simulink model "navigation"  (R2021b)
settings: Solver=VariableStepAuto  StartTime=0.0  StopTime=inf  FixedStep=0.001  RelTol=1e-3
model workspace (MAT data in the model file):
  enableTransmit = 1
undefined symbols (not defined in the file or in its folder): sampleTime
libraries: aerolibconvert2 x6, matrix_library x5, sharedutil x4, instrumentlib x1, simulink x1, aerolibutil x1
settings Model: Creator=Vladik  LastModifiedBy=Vladik

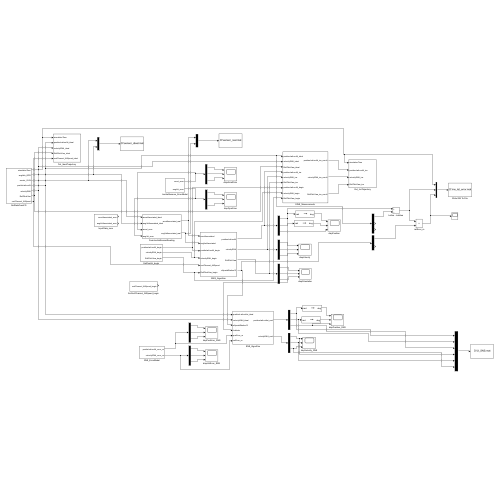
[thumbnail: Simulink's stored preview of the top-level diagram]
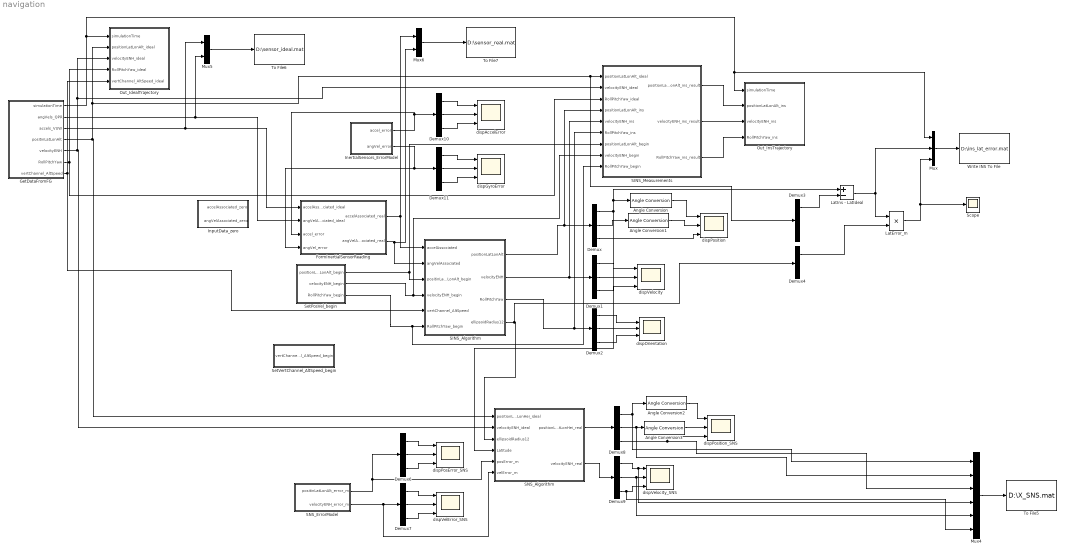
== system navigation ==
  Angle Conversion{,1..3} (4 alike) : aerolibconvert2/Angle Conversion  IU=rad  OU=deg
  Demux{,1..3,6..11} (10 alike) : Demux  Outputs=3
  Demux4 : Demux  Outputs=2
  FormInertialSensorReading : Subsystem
  GetDataFromFG : Subsystem
  InertialSensors_ErrorModel : Subsystem
  InputData_zero : Subsystem
  LatError_m : Product
  LatIns - LatIdeal : Sum  Inputs=+-
  Mux : Mux  Inputs=3
  Mux4 : Mux  Inputs=6
  Mux5 : Mux  Inputs=2
  Mux6 : Mux  Inputs=2
  Out_IdealTrajectory : Subsystem
  Out_InsTrajectory : Subsystem
  SINS_Algorithm : Subsystem
  SINS_Measurements : Subsystem
  SNS_Algorithm : Subsystem
  SNS_ErrorModel : Subsystem
  Scope : Scope
  SetPosVel_begin : Subsystem
  SetVertChannel_AltSpeed_begin : Subsystem
  To File5 : ToFile  Filename=D:\X_SNS.mat  MatrixName=x_sns
  To File6 : ToFile  Filename=D:\sensor_ideal.mat  MatrixName=sensor_ideal
  To File7 : ToFile  Filename=D:\sensor_real.mat  MatrixName=sensor_real
  Write INS To File : ToFile  Filename=D:\ins_lat_error.mat  MatrixName=ins_lat_error
  dispAccelError : Scope  NumInputPorts=3
  dispGyroError : Scope  NumInputPorts=3
  dispOrientation : Scope  NumInputPorts=3
  dispPosError_SNS : Scope  NumInputPorts=3
  dispPosition : Scope  NumInputPorts=3
  dispPosition_SNS : Scope  NumInputPorts=3
  dispVelError_SNS : Scope  NumInputPorts=3
  dispVelocity : Scope  NumInputPorts=3
  dispVelocity_SNS : Scope  NumInputPorts=3
  wires:
  Demux/1 -> LatIns - LatIdeal/1, Angle Conversion/1, SNS_Algorithm/4(Latitude)
  Demux/2 -> Angle Conversion1/1
  Demux1/1 -> dispVelocity/1
  Demux1/2 -> dispVelocity/2
  Demux1/3 -> dispVelocity/3
  Demux2/2 -> dispOrientation/2
  Demux2/1 -> dispOrientation/1
  Demux2/3 -> dispOrientation/3
  GetDataFromFG/4(positinLatLonAlt) -> Out_IdealTrajectory/2(positionLatLonAlt_ideal), Demux3/1, SINS_Measurements/1(positionLatLonAlt_ideal), SNS_Algorithm/1(positionLatLonHei_ideal)
  SINS_Algorithm/1(positionLatLonAlt) -> SINS_Measurements/4(positionLatLonAlt_ins), Demux/1
  SINS_Algorithm/2(velocityENH) -> SINS_Measurements/5(velocityENH_ins), Demux1/1
  SINS_Algorithm/3(RollPitchYaw) -> SINS_Measurements/6(RollPitchYaw_ins), Demux2/1
  SetPosVel_begin/2(velocityENH_begin) -> SINS_Measurements/8(velocityENH_begin), SINS_Algorithm/4(velocityENH_begin)
  Angle Conversion/1 -> dispPosition/1
  Angle Conversion1/1 -> dispPosition/2
  Demux6/1 -> dispPosError_SNS/1
  Demux6/2 -> dispPosError_SNS/2
  Demux6/3 -> dispPosError_SNS/3
  Demux7/1 -> dispVelError_SNS/1
  Demux7/2 -> dispVelError_SNS/2
  Demux7/3 -> dispVelError_SNS/3
  SNS_ErrorModel/2(velocityENH_error_m) -> SNS_Algorithm/6(velError_m), Demux7/1
  SNS_ErrorModel/1(positinLatLonAlt_error_m) -> SNS_Algorithm/5(posError_m), Demux6/1
  SINS_Algorithm/4(ellipsoidRadius12) -> Demux4/1, SNS_Algorithm/3(ellipsoidRadius12)
  SNS_Algorithm/1(positionLatLonHei_real) -> Demux8/1
  Demux8/3 -> Mux4/3, dispPosition_SNS/3
  Demux9/2 -> Mux4/5, dispVelocity_SNS/2
  Demux9/1 -> Mux4/4, dispVelocity_SNS/1
  Demux9/3 -> Mux4/6, dispVelocity_SNS/3
  SNS_Algorithm/2(velocityENH_real) -> Demux9/1
  Demux8/1 -> Angle Conversion2/1, Mux4/1
  Angle Conversion2/1 -> dispPosition_SNS/1
  Demux8/2 -> Mux4/2, Angle Conversion3/1
  Angle Conversion3/1 -> dispPosition_SNS/2
  Demux10/1 -> dispAccelError/1
  Demux10/2 -> dispAccelError/2
  Demux10/3 -> dispAccelError/3
  Demux11/3 -> dispGyroError/3
  Demux11/1 -> dispGyroError/1
  Demux11/2 -> dispGyroError/2
  InertialSensors_ErrorModel/1(accel_error) -> FormInertialSensorReading/3(accel_error), Demux10/1
  InertialSensors_ErrorModel/2(angVel_error) -> FormInertialSensorReading/4(angVel_error), Demux11/1
  FormInertialSensorReading/1(accelAssociated_real) -> SINS_Algorithm/1(accelAssociated), Mux6/1
  FormInertialSensorReading/2(angVelAssociated_real) -> Mux6/2, SINS_Algorithm/2(angVelAssociated)
  SetPosVel_begin/3(RollPitchYaw_begin) -> SINS_Measurements/9(RollPitchYaw_begin), SINS_Algorithm/6(RollPitchYaw_begin)
  SetPosVel_begin/1(positionLatLonAlt_begin) -> SINS_Measurements/7(positionLatLonAlt_begin), SINS_Algorithm/3(positinLatLonAlt_begin)
  GetDataFromFG/3(accels_VUW) -> Mux5/1, FormInertialSensorReading/1(accelAssociated_ideal)
  GetDataFromFG/2(angVels_QPR) -> Mux5/2, FormInertialSensorReading/2(angVelAssociated_ideal)
  GetDataFromFG/7(vertChannel_AltSpeed) -> SINS_Algorithm/5(vertChannel_AltSpeed), Out_IdealTrajectory/5(vertChannel_AltSpeed_ideal)
  GetDataFromFG/5(velocityENH) -> Out_IdealTrajectory/3(velocityENH_ideal), SINS_Measurements/2(velocityENH_ideal), SNS_Algorithm/2(velocityENH_ideal)
  Demux/3 -> dispPosition/3
  Mux4/1 -> To File5/1
  Mux5/1 -> To File6/1
  Mux6/1 -> To File7/1
  GetDataFromFG/6(RollPitchYaw) -> SINS_Measurements/3(RollPitchYaw_ideal), Out_IdealTrajectory/4(RollPitchYaw_ideal)
  SINS_Measurements/2(velocityENH_ins_result) -> Out_InsTrajectory/3(velocityENH_ins)
  SINS_Measurements/3(RollPitchYaw_ins_result) -> Out_InsTrajectory/4(RollPitchYaw_ins)
  SINS_Measurements/1(positionLatLonAlt_ins_result) -> Out_InsTrajectory/2(positionLatLonAlt_ins)
  Demux3/1 -> LatIns - LatIdeal/2
  LatIns - LatIdeal/1 -> Mux/2, LatError_m/1
  Demux4/1 -> LatError_m/2
  GetDataFromFG/1(simulationTime) -> Mux/1, Out_InsTrajectory/1(simulationTime), Out_IdealTrajectory/1(simulationTime)
  Mux/1 -> Write INS To File/1
  LatError_m/1 -> Scope/1, Mux/3

== system navigation/FormInertialSensorReading ==
  accelAssociated_ideal : Inport
  angVelAssociated_ideal : Inport  Port=2
  accel_error : Inport  Port=3
  angVel_error : Inport  Port=4
  Add : Sum
  Add1 : Sum
  accelAssociated_real : Outport
  angVelAssociated_real : Outport  Port=2
  wires:
  accelAssociated_ideal/1 -> Add/1
  accel_error/1 -> Add/2
  Add/1 -> accelAssociated_real/1
  Add1/1 -> angVelAssociated_real/1
  angVelAssociated_ideal/1 -> Add1/1
  angVel_error/1 -> Add1/2

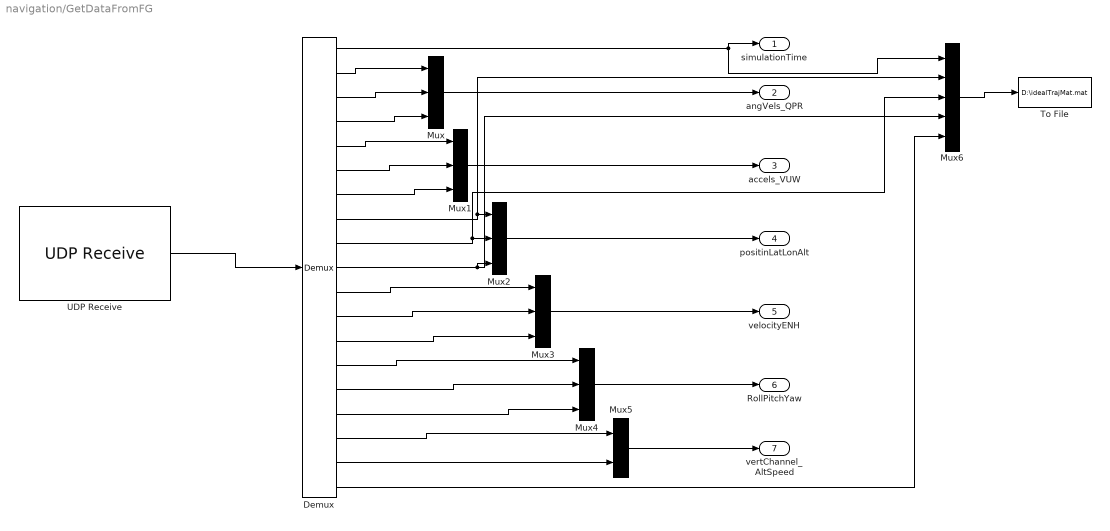
== system navigation/GetDataFromFG ==
  Demux : Demux  Outputs=19
  Mux{,1..4} (5 alike) : Mux  Inputs=3
  Mux5 : Mux  Inputs=2
  Mux6 : Mux  Inputs=5
  To File : ToFile  Filename=D:\idealTrajMat.mat  MatrixName=idealTrajData
  UDP Receive : instrumentlib/UDP Receive  Host=localhost  Port=10000  LocalPort=10000  EnablePortSharing=off  GetLatestData=off  DataSize="[1  19]"  DataType=ASCII  ASCIIFormatting=%f %f %f %f %f %f %f %f %f %f %f %f %f %f %f %f %f %f %f  Terminator=LF  ByteOrder=BigEndian  EnableBlockingMode=on  Timeout=10  SampleTime=0.01  LocalAddress=localhost
  simulationTime : Outport
  angVels_QPR : Outport  Port=2
  accels_VUW : Outport  Port=3
  positinLatLonAlt : Outport  Port=4
  velocityENH : Outport  Port=5
  RollPitchYaw : Outport  Port=6
  vertChannel_AltSpeed : Outport  Port=7
  wires:
  UDP Receive/1 -> Demux/1
  Demux/2 -> Mux/1
  Demux/3 -> Mux/2
  Demux/4 -> Mux/3
  Demux/5 -> Mux1/1
  Demux/6 -> Mux1/2
  Demux/7 -> Mux1/3
  Demux/8 -> Mux6/2, Mux2/1
  Demux/9 -> Mux6/3, Mux2/2
  Demux/10 -> Mux2/3, Mux6/4
  Mux/1 -> angVels_QPR/1
  Mux1/1 -> accels_VUW/1
  Mux2/1 -> positinLatLonAlt/1
  Demux/11 -> Mux3/1
  Demux/12 -> Mux3/2
  Demux/13 -> Mux3/3
  Mux3/1 -> velocityENH/1
  Demux/14 -> Mux4/1
  Demux/15 -> Mux4/2
  Demux/16 -> Mux4/3
  Mux4/1 -> RollPitchYaw/1
  Demux/17 -> Mux5/1
  Demux/18 -> Mux5/2
  Mux5/1 -> vertChannel_AltSpeed/1
  Demux/1 -> simulationTime/1, Mux6/1
  Mux6/1 -> To File/1
  Demux/19 -> Mux6/5

== system navigation/InertialSensors_ErrorModel ==
  Add{,1..5} (6 alike) : Sum
  Mux : Mux  Inputs=3
  Mux1 : Mux  Inputs=3
  Ramp : simulink/Sources/Ramp  slope=0.15*pi/180/3600  start=0  InitialOutput=0
  accelNoise : RandomNumber  Mean=1e-6  Variance=0  SampleTime=1
  accelZeroOffset : Constant  Value=0.005
  gyroNoise : RandomNumber  Mean=(0.1*pi/180/3600)^2  Variance=0  SampleTime=1
  accel_error : Outport
  angVel_error : Outport  Port=2
  wires:
  gyroNoise/1 -> Add/2, Add5/2, Add4/2
  accelZeroOffset/1 -> Add2/1, Add3/1, Add1/1
  accelNoise/1 -> Add3/2, Add2/2, Add1/2
  Add1/1 -> Mux/2
  Mux/1 -> accel_error/1
  Mux1/1 -> angVel_error/1
  Add2/1 -> Mux/1
  Add3/1 -> Mux/3
  Ramp/1 -> Add5/1, Add4/1, Add/1
  Add4/1 -> Mux1/2
  Add/1 -> Mux1/1
  Add5/1 -> Mux1/3

== system navigation/InputData_zero ==
  Constant : Constant  Value=1e-5
  Constant1 : Constant  Value=1e-5
  Constant2 : Constant  Value=0.1
  Mux : Mux  Inputs=3
  Mux1 : Mux  Inputs=3
  accelAssociated_zero : Outport
  angVelAssociated_zero : Outport  Port=2
  wires:
  Constant/1 -> Mux1/2, Mux1/3, Mux1/1, Mux/2
  Mux/1 -> accelAssociated_zero/1
  Mux1/1 -> angVelAssociated_zero/1
  Constant1/1 -> Mux/3
  Constant2/1 -> Mux/1

== system navigation/Out_IdealTrajectory ==
  simulationTime : Inport
  positionLatLonAlt_ideal : Inport  Port=2
  velocityENH_ideal : Inport  Port=3
  RollPitchYaw_ideal : Inport  Port=4
  vertChannel_AltSpeed_ideal : Inport  Port=5
  Demux3 : Demux  Outputs=3
  Demux4 : Demux  Outputs=3
  Demux5 : Demux  Outputs=3
  Vector Concatenate2 : Concatenate  NumInputs=5  Mode=Multidimensional array
  Write Ideal To File : ToFile  Filename=D:\x_ideal.mat  MatrixName=x_ideal
  dispOrientationIdeal : Scope  NumInputPorts=3
  dispPositionIdeal : Scope  NumInputPorts=3
  dispVelocityIdeal : Scope  NumInputPorts=3
  wires:
  simulationTime/1 -> Vector Concatenate2/1
  positionLatLonAlt_ideal/1 -> Demux3/1, Vector Concatenate2/2
  RollPitchYaw_ideal/1 -> Demux5/1, Vector Concatenate2/4
  vertChannel_AltSpeed_ideal/1 -> Vector Concatenate2/5
  Vector Concatenate2/1 -> Write Ideal To File/1
  Demux3/2 -> dispPositionIdeal/2
  Demux3/3 -> dispPositionIdeal/3
  Demux3/1 -> dispPositionIdeal/1
  velocityENH_ideal/1 -> Demux4/1, Vector Concatenate2/3
  Demux4/1 -> dispVelocityIdeal/1
  Demux4/2 -> dispVelocityIdeal/2
  Demux4/3 -> dispVelocityIdeal/3
  Demux5/3 -> dispOrientationIdeal/3
  Demux5/2 -> dispOrientationIdeal/2
  Demux5/1 -> dispOrientationIdeal/1

== system navigation/Out_InsTrajectory ==
  simulationTime : Inport
  positionLatLonAlt_ins : Inport  Port=2
  velocityENH_ins : Inport  Port=3
  RollPitchYaw_ins : Inport  Port=4
  Demux3 : Demux  Outputs=3
  Demux4 : Demux  Outputs=3
  Demux5 : Demux  Outputs=3
  Vector Concatenate2 : Concatenate  NumInputs=4  Mode=Multidimensional array
  Write INS To File : ToFile  Filename=D:\x_ins.mat  MatrixName=x_ins
  dispOrientationINS : Scope  NumInputPorts=3
  dispPositionINS : Scope  NumInputPorts=3
  dispVelocityINS : Scope  NumInputPorts=3
  wires:
  simulationTime/1 -> Vector Concatenate2/1
  positionLatLonAlt_ins/1 -> Demux3/1, Vector Concatenate2/2
  RollPitchYaw_ins/1 -> Demux5/1, Vector Concatenate2/4
  Vector Concatenate2/1 -> Write INS To File/1
  Demux3/2 -> dispPositionINS/2
  Demux3/3 -> dispPositionINS/3
  Demux3/1 -> dispPositionINS/1
  velocityENH_ins/1 -> Demux4/1, Vector Concatenate2/3
  Demux4/1 -> dispVelocityINS/1
  Demux4/2 -> dispVelocityINS/2
  Demux4/3 -> dispVelocityINS/3
  Demux5/3 -> dispOrientationINS/3
  Demux5/2 -> dispOrientationINS/2
  Demux5/1 -> dispOrientationINS/1

== system navigation/SINS_Algorithm ==
  accelAssociated : Inport
  angVelAssociated : Inport  Port=2
  positinLatLonAlt_begin : Inport  Port=3
  velocityENH_begin : Inport  Port=4
  vertChannel_AltSpeed : Inport  Port=5
  RollPitchYaw_begin : Inport  Port=6
  CalculateAccelerationsXYZ : Subsystem
  GetC_begin : Subsystem  Commented=on
  GetC_begin_easy : Subsystem
  NavigationAlgorithm : Subsystem
  OrientationAlgorithm : Subsystem
  U_earth : Constant  Value=7.29212e-5
  removeVelocityH : Subsystem
  positionLatLonAlt : Outport
  velocityENH : Outport  Port=2
  RollPitchYaw : Outport  Port=3
  ellipsoidRadius12 : Outport  Port=4
  wires:
  accelAssociated/1 -> CalculateAccelerationsXYZ/1(accelerationAssociated)
  OrientationAlgorithm/1(C_assoc_norm) -> CalculateAccelerationsXYZ/2(C_accoc_norm)
  angVelAssociated/1 -> OrientationAlgorithm/1(angVel_inertial_assoc)
  NavigationAlgorithm/3(angVelNorm_matrix_3x3) -> OrientationAlgorithm/2(angVelNorm_matrix)
  NavigationAlgorithm/1(positionLatLonAlt) -> positionLatLonAlt/1
  NavigationAlgorithm/2(velocityENH) -> velocityENH/1
  OrientationAlgorithm/2(RollPitchYaw) -> RollPitchYaw/1
  positinLatLonAlt_begin/1 -> NavigationAlgorithm/2(positionLatLonAlt_begin)
  U_earth/1 -> NavigationAlgorithm/4(U_earth)
  vertChannel_AltSpeed/1 -> NavigationAlgorithm/5(vertChannel_AltSpeed)
  NavigationAlgorithm/4(ellipsoidRadius12) -> ellipsoidRadius12/1
  velocityENH_begin/1 -> removeVelocityH/1(velocityENH_begin)
  removeVelocityH/1(velocityEN_begin) -> NavigationAlgorithm/3(velocityEN_begin)
  RollPitchYaw_begin/1 -> GetC_begin_easy/1(RollPitchYaw_begin)
  GetC_begin_easy/1(C_assoc_norm_begin) -> OrientationAlgorithm/3(C_assoc_norm_begin)
  CalculateAccelerationsXYZ/1(accelerationXYZ) -> NavigationAlgorithm/1(accelerationXYZ)

== system navigation/SINS_Measurements ==
  positionLatLonAlt_ideal : Inport
  velocityENH_ideal : Inport  Port=2
  RollPitchYaw_ideal : Inport  Port=3
  positionLatLonAlt_ins : Inport  Port=4
  velocityENH_ins : Inport  Port=5
  RollPitchYaw_ins : Inport  Port=6
  positionLatLonAlt_begin : Inport  Port=7
  velocityENH_begin : Inport  Port=8
  RollPitchYaw_begin : Inport  Port=9
  Subtract1 : Sum  Inputs=++-
  Subtract2 : Sum  Inputs=++-
  Subtract3 : Sum  Inputs=++-
  positionLatLonAlt_ins_result : Outport
  velocityENH_ins_result : Outport  Port=2
  RollPitchYaw_ins_result : Outport  Port=3
  wires:
  positionLatLonAlt_ideal/1 -> Subtract3/1
  positionLatLonAlt_ins/1 -> Subtract3/2
  positionLatLonAlt_begin/1 -> Subtract3/3
  velocityENH_ideal/1 -> Subtract1/1
  velocityENH_ins/1 -> Subtract1/2
  velocityENH_begin/1 -> Subtract1/3
  RollPitchYaw_ideal/1 -> Subtract2/1
  RollPitchYaw_ins/1 -> Subtract2/2
  RollPitchYaw_begin/1 -> Subtract2/3
  Subtract3/1 -> positionLatLonAlt_ins_result/1
  Subtract1/1 -> velocityENH_ins_result/1
  Subtract2/1 -> RollPitchYaw_ins_result/1

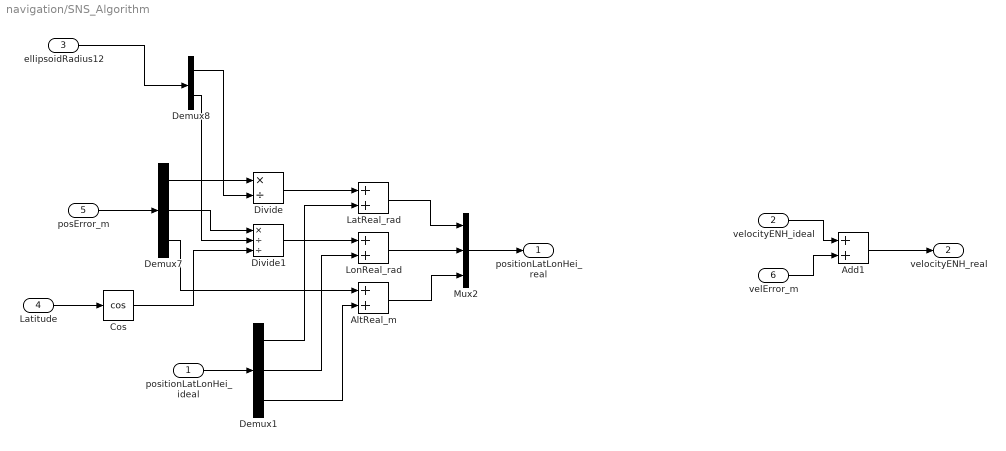
== system navigation/SNS_Algorithm ==
  positionLatLonHei_ideal : Inport
  velocityENH_ideal : Inport  Port=2
  ellipsoidRadius12 : Inport  Port=3
  Latitude : Inport  Port=4
  posError_m : Inport  Port=5
  velError_m : Inport  Port=6
  Add1 : Sum
  AltReal_m : Sum
  Cos : Trigonometry  Operator=cos
  Demux1 : Demux  Outputs=3
  Demux7 : Demux  Outputs=3
  Demux8 : Demux  Outputs=2
  Divide : Product  Inputs=*/
  Divide1 : Product  Inputs=*//
  LatReal_rad : Sum
  LonReal_rad : Sum
  Mux2 : Mux  Inputs=3
  positionLatLonHei_real : Outport
  velocityENH_real : Outport  Port=2
  wires:
  Divide1/1 -> LonReal_rad/1
  Divide/1 -> LatReal_rad/1
  ellipsoidRadius12/1 -> Demux8/1
  posError_m/1 -> Demux7/1
  Demux7/1 -> Divide/1
  Demux8/1 -> Divide/2
  Demux7/2 -> Divide1/1
  Demux8/2 -> Divide1/2
  Latitude/1 -> Cos/1
  Cos/1 -> Divide1/3
  positionLatLonHei_ideal/1 -> Demux1/1
  Demux1/1 -> LatReal_rad/2
  Demux1/2 -> LonReal_rad/2
  Demux7/3 -> AltReal_m/1
  Demux1/3 -> AltReal_m/2
  LonReal_rad/1 -> Mux2/2
  LatReal_rad/1 -> Mux2/1
  AltReal_m/1 -> Mux2/3
  Mux2/1 -> positionLatLonHei_real/1
  velocityENH_ideal/1 -> Add1/1
  velError_m/1 -> Add1/2
  Add1/1 -> velocityENH_real/1

== system navigation/SNS_ErrorModel ==
  AltError_m : RandomNumber  Variance=225  SampleTime=sampleTime
  LatError_m : RandomNumber  Variance=225  SampleTime=sampleTime
  LonError_m : RandomNumber  Variance=225  SampleTime=sampleTime
  Mux : Mux  Inputs=3
  Mux1 : Mux  Inputs=3
  VelE_error_m : RandomNumber  Variance=0.01  SampleTime=sampleTime
  VelH_error_m : RandomNumber  Variance=0.01  SampleTime=sampleTime
  VelN_error_m : RandomNumber  Variance=0.01  SampleTime=sampleTime
  positinLatLonAlt_error_m : Outport
  velocityENH_error_m : Outport  Port=2
  wires:
  LonError_m/1 -> Mux/2
  LatError_m/1 -> Mux/1
  AltError_m/1 -> Mux/3
  Mux/1 -> positinLatLonAlt_error_m/1
  VelN_error_m/1 -> Mux1/2
  VelE_error_m/1 -> Mux1/1
  VelH_error_m/1 -> Mux1/3
  Mux1/1 -> velocityENH_error_m/1

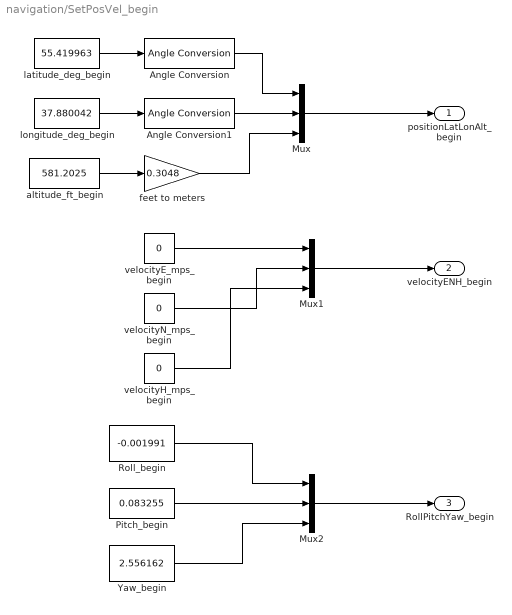
== system navigation/SetPosVel_begin ==
  Angle Conversion : aerolibconvert2/Angle Conversion  IU=deg  OU=rad
  Angle Conversion1 : aerolibconvert2/Angle Conversion  IU=deg  OU=rad
  Mux : Mux  Inputs=3
  Mux1 : Mux  Inputs=3
  Mux2 : Mux  Inputs=3
  Pitch_begin : Constant  Value=0.083255
  Roll_begin : Constant  Value=-0.001991
  Yaw_begin : Constant  Value=2.556162
  altitude_ft_begin : Constant  Value=581.2025
  feet to meters : Gain  Gain=0.3048
  latitude_deg_begin : Constant  Value=55.419963
  longitude_deg_begin : Constant  Value=37.880042
  velocityE_mps_begin : Constant  Value=0
  velocityH_mps_begin : Constant  Value=0
  velocityN_mps_begin : Constant  Value=0
  positionLatLonAlt_begin : Outport
  velocityENH_begin : Outport  Port=2
  RollPitchYaw_begin : Outport  Port=3
  wires:
  altitude_ft_begin/1 -> feet to meters/1
  latitude_deg_begin/1 -> Angle Conversion/1
  Mux1/1 -> velocityENH_begin/1
  velocityE_mps_begin/1 -> Mux1/1
  Angle Conversion1/1 -> Mux/2
  feet to meters/1 -> Mux/3
  velocityN_mps_begin/1 -> Mux1/2
  longitude_deg_begin/1 -> Angle Conversion1/1
  Angle Conversion/1 -> Mux/1
  Mux/1 -> positionLatLonAlt_begin/1
  velocityH_mps_begin/1 -> Mux1/3
  Yaw_begin/1 -> Mux2/3
  Pitch_begin/1 -> Mux2/2
  Roll_begin/1 -> Mux2/1
  Mux2/1 -> RollPitchYaw_begin/1

== system navigation/SetVertChannel_AltSpeed_begin ==
  Mux : Mux  Inputs=2
  altitude_ft_begin : Constant  Value=497.4182917
  feet to meters : Gain  Gain=0.3048
  velocityH_mps_begin : Constant  Value=0
  vertChannel_AltSpeed_begin : Outport
  wires:
  velocityH_mps_begin/1 -> Mux/2
  feet to meters/1 -> Mux/1
  altitude_ft_begin/1 -> feet to meters/1
  Mux/1 -> vertChannel_AltSpeed_begin/1

== system navigation/SINS_Algorithm/CalculateAccelerationsXYZ ==
  accelerationAssociated : Inport
  C_accoc_norm : Inport  Port=2
  Product : Product  Multiplication=Matrix(*)
  accelerationXYZ : Outport
  wires:
  accelerationAssociated/1 -> Product/2
  Product/1 -> accelerationXYZ/1
  C_accoc_norm/1 -> Product/1

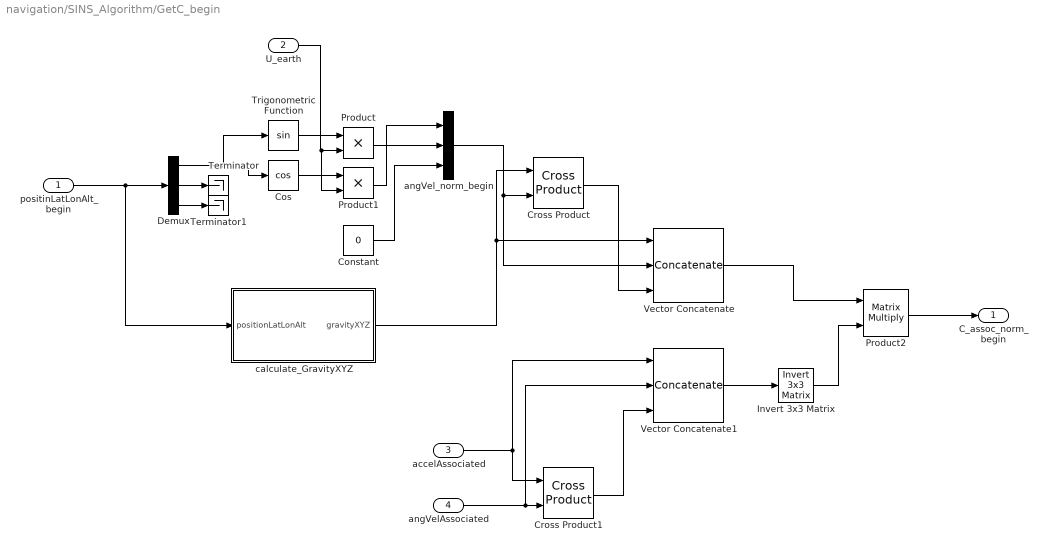
== system navigation/SINS_Algorithm/GetC_begin ==
  positinLatLonAlt_begin : Inport
  U_earth : Inport  Port=2
  accelAssociated : Inport  Port=3
  angVelAssociated : Inport  Port=4
  Constant : Constant  Value=0
  Cos : Trigonometry  Operator=cos
  Cross Product : matrix_library/Cross Product
      settings: SourceProductBaseCode=SL
  Cross Product1 : matrix_library/Cross Product
      settings: SourceProductBaseCode=SL
  Demux : Demux  Outputs=3
  Invert 3x3 Matrix : aerolibutil/Invert  3x3 Matrix
  Product : Product
  Product1 : Product
  Product2 : Product  Multiplication=Matrix(*)
  Terminator : Terminator
  Terminator1 : Terminator
  Trigonometric Function : Trigonometry
  Vector Concatenate : Concatenate  NumInputs=3  Mode=Multidimensional array  ConcatenateDimension=2
  Vector Concatenate1 : Concatenate  NumInputs=3  Mode=Multidimensional array  ConcatenateDimension=2
  angVel_norm_begin : Mux  Inputs=3
  calculate_GravityXYZ : Subsystem
  C_assoc_norm_begin : Outport
  wires:
  Trigonometric Function/1 -> Product/1
  Demux/1 -> Cos/1, Trigonometric Function/1
  Cos/1 -> Product1/1
  Constant/1 -> angVel_norm_begin/3
  Product/1 -> angVel_norm_begin/2
  Product1/1 -> angVel_norm_begin/1
  Demux/3 -> Terminator1/1
  Demux/2 -> Terminator/1
  calculate_GravityXYZ/1(gravityXYZ) -> Vector Concatenate/1, Cross Product/1
  angVel_norm_begin/1 -> Vector Concatenate/2, Cross Product/2
  positinLatLonAlt_begin/1 -> calculate_GravityXYZ/1(positionLatLonAlt), Demux/1
  U_earth/1 -> Product1/2, Product/2
  Cross Product/1 -> Vector Concatenate/3
  accelAssociated/1 -> Vector Concatenate1/1, Cross Product1/1
  angVelAssociated/1 -> Vector Concatenate1/2, Cross Product1/2
  Cross Product1/1 -> Vector Concatenate1/3
  Vector Concatenate1/1 -> Invert 3x3 Matrix/1
  Vector Concatenate/1 -> Product2/1
  Invert 3x3 Matrix/1 -> Product2/2
  Product2/1 -> C_assoc_norm_begin/1

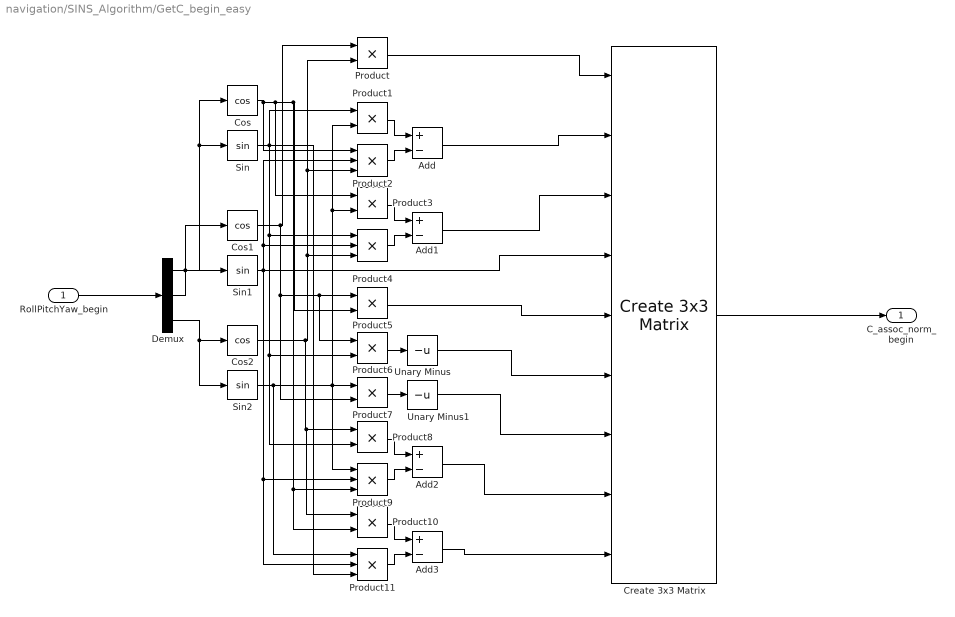
== system navigation/SINS_Algorithm/GetC_begin_easy ==
  RollPitchYaw_begin : Inport
  Add{,1..3} (4 alike) : Sum  Inputs=+-
  Cos : Trigonometry  Operator=cos
  Cos1 : Trigonometry  Operator=cos
  Cos2 : Trigonometry  Operator=cos
  Create 3x3 Matrix : sharedutil/Create 3x3 Matrix  aMode=aMode
      settings: SourceProductBaseCode=AE,PW,DR,MT,UV,VE
  Demux : Demux  Outputs=3
  Product{,1,3,5..8,10} (8 alike) : Product
  Product{2,4,9,11} (4 alike) : Product  Inputs=3
  Sin : Trigonometry
  Sin1 : Trigonometry
  Sin2 : Trigonometry
  Unary Minus : UnaryMinus
  Unary Minus1 : UnaryMinus
  C_assoc_norm_begin : Outport
  wires:
  RollPitchYaw_begin/1 -> Demux/1
  Demux/1 -> Sin/1, Cos/1
  Demux/2 -> Sin1/1, Cos1/1
  Demux/3 -> Sin2/1, Cos2/1
  Cos1/1 -> Product7/2, Product6/1, Product5/1, Product/1
  Sin2/1 -> Product11/1, Product9/1, Product7/1, Product3/2, Product1/2
  Sin/1 -> Product11/3, Product8/2, Product6/2, Product4/1, Product1/1
  Sin1/1 -> Product11/2, Product9/2, Create 3x3 Matrix/4, Product4/2, Product2/2
  Cos/1 -> Product10/2, Product9/3, Product5/2, Product3/1, Product2/1
  Product1/1 -> Add/1
  Product2/1 -> Add/2
  Product/1 -> Create 3x3 Matrix/1
  Add/1 -> Create 3x3 Matrix/2
  Product4/1 -> Add1/2
  Product3/1 -> Add1/1
  Add1/1 -> Create 3x3 Matrix/3
  Product5/1 -> Create 3x3 Matrix/5
  Product6/1 -> Unary Minus/1
  Unary Minus/1 -> Create 3x3 Matrix/6
  Product7/1 -> Unary Minus1/1
  Cos2/1 -> Product10/1, Product8/1, Product4/3, Product2/3, Product/2
  Unary Minus1/1 -> Create 3x3 Matrix/7
  Product8/1 -> Add2/1
  Product9/1 -> Add2/2
  Add2/1 -> Create 3x3 Matrix/8
  Product11/1 -> Add3/2
  Product10/1 -> Add3/1
  Add3/1 -> Create 3x3 Matrix/9
  Create 3x3 Matrix/1 -> C_assoc_norm_begin/1

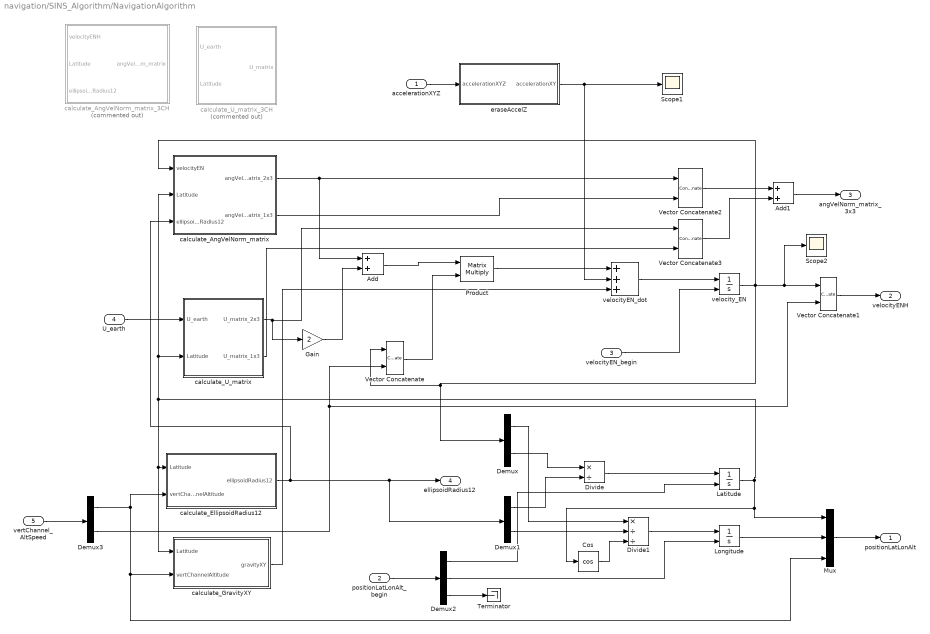
== system navigation/SINS_Algorithm/NavigationAlgorithm ==
  accelerationXYZ : Inport
  positionLatLonAlt_begin : Inport  Port=2
  velocityEN_begin : Inport  Port=3
  U_earth : Inport  Port=4
  vertChannel_AltSpeed : Inport  Port=5
  Add : Sum
  Add1 : Sum
  Cos : Trigonometry  Operator=cos
  Demux : Demux  Outputs=2
  Demux1 : Demux  Outputs=2
  Demux2 : Demux  Outputs=3
  Demux3 : Demux  Outputs=2
  Divide : Product  Inputs=*/
  Divide1 : Product  Inputs=*//
  Gain : Gain  Gain=2
  Latitude : Integrator  InitialConditionSource=external
  Longitude : Integrator  InitialConditionSource=external
  Mux : Mux  Inputs=3
  Product : Product  Multiplication=Matrix(*)
  Scope1 : Scope
  Scope2 : Scope
  Terminator : Terminator
  Vector Concatenate{,1..3} (4 alike) : Concatenate  Mode=Multidimensional array
  calculate_AngVelNorm_matrix : Subsystem
  calculate_AngVelNorm_matrix_3CH : Subsystem  Commented=on
  calculate_EllipsoidRadius12 : Subsystem
  calculate_GravityXY : Subsystem
  calculate_U_matrix : Subsystem
  calculate_U_matrix_3CH : Subsystem  Commented=on
  eraseAccelZ : Subsystem
  velocityEN_dot : Sum  Inputs=+++
  velocity_EN : Integrator  InitialConditionSource=external  InitialCondition=[0; 0; 0]
  positionLatLonAlt : Outport
  velocityENH : Outport  Port=2
  angVelNorm_matrix_3x3 : Outport  Port=3
  ellipsoidRadius12 : Outport  Port=4
  wires:
  calculate_U_matrix/1(U_matrix_2x3) -> Vector Concatenate3/1, Gain/1
  calculate_AngVelNorm_matrix/1(angVelNorm_matrix_2x3) -> Vector Concatenate2/1, Add/1
  Gain/1 -> Add/2
  Add/1 -> Product/1
  Product/1 -> velocityEN_dot/1
  velocityEN_dot/1 -> velocity_EN/1
  Divide/1 -> Latitude/1
  Demux/2 -> Divide/1
  Demux1/1 -> Divide/2
  Latitude/1 -> calculate_GravityXY/1(Latitude), calculate_EllipsoidRadius12/1(Latitude), calculate_U_matrix/2(Latitude), calculate_AngVelNorm_matrix/2(Latitude), Mux/1, Cos/1
  Divide1/1 -> Longitude/1
  Demux/1 -> Divide1/1
  Demux1/2 -> Divide1/2
  Cos/1 -> Divide1/3
  Longitude/1 -> Mux/2
  Demux3/1 -> Mux/3, calculate_GravityXY/2(vertChannelAltitude), calculate_EllipsoidRadius12/2(vertChannelAltitude)
  calculate_EllipsoidRadius12/1(ellipsoidRadius12) -> calculate_AngVelNorm_matrix/3(ellipsoidRadius12), ellipsoidRadius12/1, Demux1/1
  U_earth/1 -> calculate_U_matrix/1(U_earth)
  Mux/1 -> positionLatLonAlt/1
  velocity_EN/1 -> Scope2/1, Vector Concatenate1/1, calculate_AngVelNorm_matrix/1(velocityEN), Vector Concatenate/1, Demux/1
  calculate_GravityXY/1(gravityXY) -> velocityEN_dot/3
  positionLatLonAlt_begin/1 -> Demux2/1
  Demux2/1 -> Latitude/2
  Demux2/2 -> Longitude/2
  velocityEN_begin/1 -> velocity_EN/2
  vertChannel_AltSpeed/1 -> Demux3/1
  Demux3/2 -> Vector Concatenate1/2, Vector Concatenate/2
  Vector Concatenate/1 -> Product/2
  Vector Concatenate1/1 -> velocityENH/1
  calculate_AngVelNorm_matrix/2(angVelNorm_matrix_1x3) -> Vector Concatenate2/2
  accelerationXYZ/1 -> eraseAccelZ/1(accelerationXYZ)
  eraseAccelZ/1(accelerationXY) -> Scope1/1, velocityEN_dot/2
  Demux2/3 -> Terminator/1
  calculate_U_matrix/2(U_matrix_1x3) -> Vector Concatenate3/2
  Vector Concatenate2/1 -> Add1/1
  Vector Concatenate3/1 -> Add1/2
  Add1/1 -> angVelNorm_matrix_3x3/1

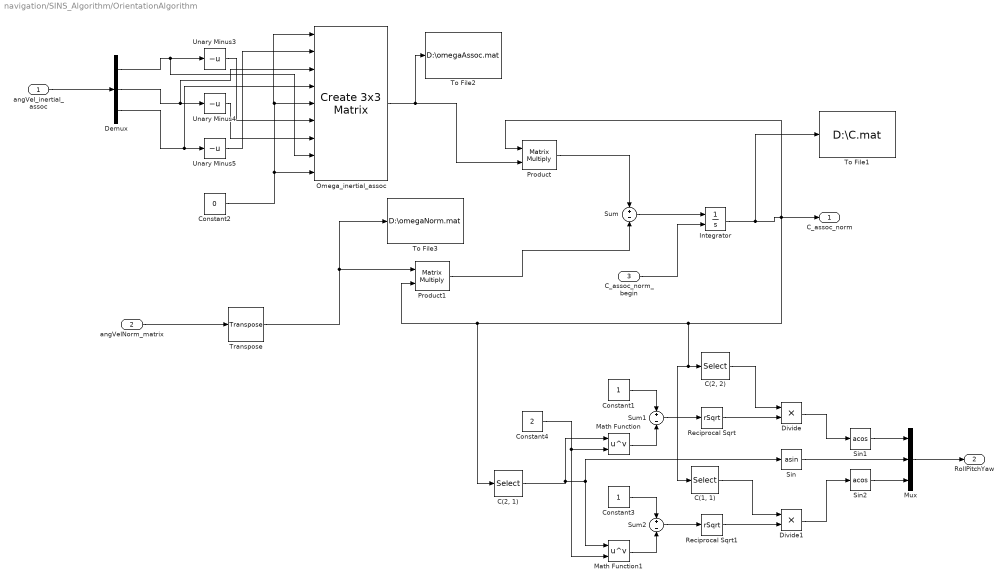
== system navigation/SINS_Algorithm/OrientationAlgorithm ==
  angVel_inertial_assoc : Inport
  angVelNorm_matrix : Inport  Port=2
  C_assoc_norm_begin : Inport  Port=3
  "C(1, 1)" : Selector  NumberOfDimensions=2  InputPortWidth=3  IndexOptions=Index vector (dialog),Index vector (dialog)  Indices=1,1  OutputSizes=1,1
  "C(2, 1)" : Selector  NumberOfDimensions=2  InputPortWidth=3  IndexOptions=Index vector (dialog),Index vector (dialog)  Indices=2,1  OutputSizes=1,1
  "C(2, 2)" : Selector  NumberOfDimensions=2  InputPortWidth=3  IndexOptions=Index vector (dialog),Index vector (dialog)  Indices=2,2  OutputSizes=1,1
  Constant1 : Constant
  Constant2 : Constant  Value=0
  Constant3 : Constant
  Constant4 : Constant  Value=2
  Demux : Demux  Outputs=3
  Divide : Product  Inputs=**
  Divide1 : Product  Inputs=**
  Integrator : Integrator  InitialConditionSource=external  InitialCondition=[0, 0, 0; 0, 0, 0; 0, 0, 0]
  Math Function : Math  Operator=pow  SaturateOnIntegerOverflow=on
  Math Function1 : Math  Operator=pow  SaturateOnIntegerOverflow=on
  Mux : Mux  Inputs=3
  Omega_inertial_assoc : sharedutil/Create 3x3 Matrix  aMode=aMode
      settings: SourceProductBaseCode=AE,PW,DR,MT,UV,VE
  Product : Product  Multiplication=Matrix(*)
  Product1 : Product  Multiplication=Matrix(*)
  Reciprocal Sqrt : Sqrt  Operator=rSqrt  SaturateOnIntegerOverflow=on
  Reciprocal Sqrt1 : Sqrt  Operator=rSqrt  SaturateOnIntegerOverflow=on
  Sin : Trigonometry  Operator=asin
  Sin1 : Trigonometry  Operator=acos
  Sin2 : Trigonometry  Operator=acos
  Sum : Sum  Inputs=+-
  Sum1 : Sum  Inputs=+-
  Sum2 : Sum  Inputs=+-
  To File1 : ToFile  Filename=D:\C.mat  MatrixName=C  SaveFormat=Timeseries
  To File2 : ToFile  Filename=D:\omegaAssoc.mat  MatrixName=omegaAssoc  SaveFormat=Timeseries
  To File3 : ToFile  Filename=D:\omegaNorm.mat  MatrixName=omegaNorm  SaveFormat=Timeseries
  Transpose : matrix_library/Transpose
      settings: SourceProductBaseCode=SL
  Unary Minus3 : UnaryMinus
  Unary Minus4 : UnaryMinus
  Unary Minus5 : UnaryMinus
  C_assoc_norm : Outport
  RollPitchYaw : Outport  Port=2
  wires:
  angVel_inertial_assoc/1 -> Demux/1
  angVelNorm_matrix/1 -> Transpose/1
  Sum/1 -> Integrator/1
  Transpose/1 -> To File3/1, Product1/1
  Omega_inertial_assoc/1 -> To File2/1, Product/2
  Product/1 -> Sum/1
  Product1/1 -> Sum/2
  Reciprocal Sqrt/1 -> Divide/2
  Math Function/1 -> Sum1/2
  Mux/1 -> RollPitchYaw/1
  "C(2, 2)"/1 -> Divide/1
  Divide1/1 -> Sin2/1
  Constant3/1 -> Sum2/1
  "C(2, 1)"/1 -> Math Function/1, Math Function1/1, Sin/1
  Divide/1 -> Sin1/1
  Sum1/1 -> Reciprocal Sqrt/1
  Constant1/1 -> Sum1/1
  Constant4/1 -> Math Function1/2, Math Function/2
  Sum2/1 -> Reciprocal Sqrt1/1
  Reciprocal Sqrt1/1 -> Divide1/2
  Sin/1 -> Mux/2
  Sin1/1 -> Mux/1
  Sin2/1 -> Mux/3
  "C(1, 1)"/1 -> Divide1/1
  Math Function1/1 -> Sum2/2
  C_assoc_norm_begin/1 -> Integrator/2
  Integrator/1 -> To File1/1, "C(2, 2)"/1, "C(1, 1)"/1, "C(2, 1)"/1, Product1/2, Product/1, C_assoc_norm/1
  Unary Minus5/1 -> Omega_inertial_assoc/2
  Unary Minus3/1 -> Omega_inertial_assoc/6
  Constant2/1 -> Omega_inertial_assoc/1, Omega_inertial_assoc/5, Omega_inertial_assoc/9
  Unary Minus4/1 -> Omega_inertial_assoc/7
  Demux/3 -> Omega_inertial_assoc/4, Unary Minus5/1
  Demux/2 -> Omega_inertial_assoc/3, Unary Minus4/1
  Demux/1 -> Omega_inertial_assoc/8, Unary Minus3/1

== system navigation/SINS_Algorithm/removeVelocityH ==
  velocityENH_begin : Inport
  Demux : Demux  Outputs=3
  Mux : Mux  Inputs=2
  Terminator : Terminator
  velocityEN_begin : Outport
  wires:
  velocityENH_begin/1 -> Demux/1
  Demux/1 -> Mux/1
  Demux/2 -> Mux/2
  Mux/1 -> velocityEN_begin/1
  Demux/3 -> Terminator/1

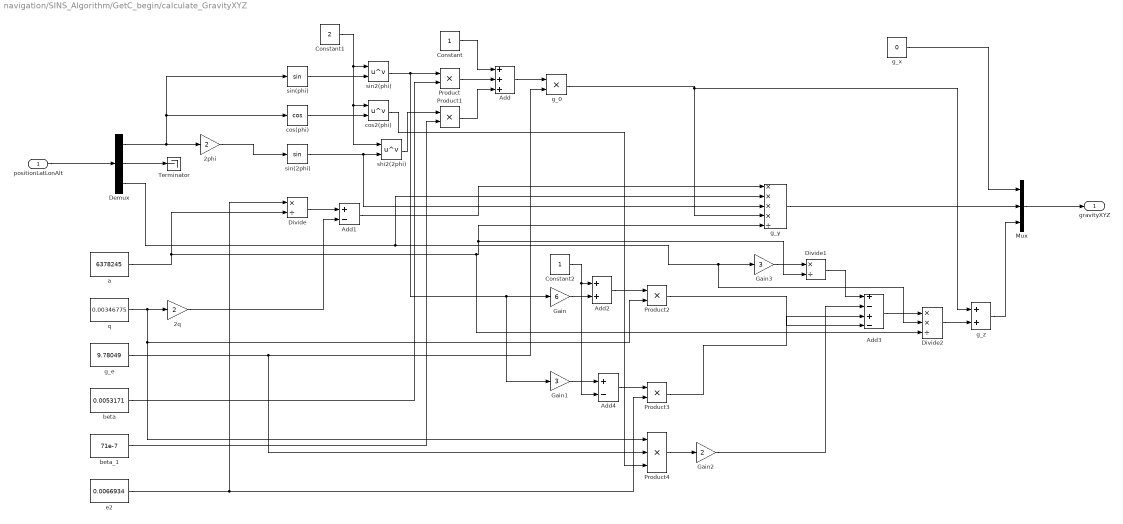
== system navigation/SINS_Algorithm/GetC_begin/calculate_GravityXYZ ==
  positionLatLonAlt : Inport
  2phi : Gain  Gain=2
  2q : Gain  Gain=2
  Add : Sum  Inputs=+++
  Add1 : Sum  Inputs=+-
  Add2 : Sum
  Add3 : Sum  Inputs=+-+-
  Add4 : Sum  Inputs=+-
  Constant : Constant
  Constant1 : Constant  Value=2
  Constant2 : Constant
  Demux : Demux  Outputs=3
  Divide : Product  Inputs=*/
  Divide1 : Product  Inputs=*/
  Divide2 : Product  Inputs=**/
  Gain : Gain  Gain=6
  Gain1 : Gain  Gain=3
  Gain2 : Gain  Gain=2
  Gain3 : Gain  Gain=3
  Mux : Mux  Inputs=3
  Product{,1..3} (4 alike) : Product
  Product4 : Product  Inputs=3
  Terminator : Terminator
  a : Constant  Value=6378245
  beta : Constant  Value=0.0053171
  beta_1 : Constant  Value=71e-7
  cos(phi) : Trigonometry  Operator=cos
  cos2(phi) : Math  Operator=pow  SaturateOnIntegerOverflow=on
  e2 : Constant  Value=0.0066934
  g_0 : Product
  g_e : Constant  Value=9.78049
  g_x : Constant  Value=0
  g_y : Product  Inputs=****/
  g_z : Sum
  q : Constant  Value=0.00346775
  shi2(2phi) : Math  Operator=pow  SaturateOnIntegerOverflow=on
  sin(2phi) : Trigonometry
  sin(phi) : Trigonometry
  sin2(phi) : Math  Operator=pow  SaturateOnIntegerOverflow=on
  gravityXYZ : Outport
  wires:
  positionLatLonAlt/1 -> Demux/1
  Demux/2 -> Terminator/1
  Mux/1 -> gravityXYZ/1
  Demux/1 -> cos(phi)/1, sin(phi)/1, 2phi/1
  2phi/1 -> sin(2phi)/1
  sin(phi)/1 -> sin2(phi)/2
  Constant1/1 -> cos2(phi)/1, shi2(2phi)/1, sin2(phi)/1
  sin(2phi)/1 -> g_y/3, shi2(2phi)/2
  beta/1 -> Product/2
  sin2(phi)/1 -> Gain1/1, Gain/1, Product/1
  shi2(2phi)/1 -> Product1/1
  beta_1/1 -> Product1/2
  Product/1 -> Add/2
  Constant/1 -> Add/1
  Product1/1 -> Add/3
  Add/1 -> g_0/1
  g_e/1 -> Product4/2, g_0/2
  e2/1 -> Product3/2, Divide/1
  a/1 -> Divide2/3, Divide1/2, g_y/5, Divide/2
  Divide/1 -> Add1/1
  q/1 -> Product4/1, Product2/2, 2q/1
  2q/1 -> Add1/2
  Add1/1 -> g_y/1
  Demux/3 -> g_y/2, Divide2/2, Gain3/1
  g_0/1 -> g_z/1, g_y/4
  g_y/1 -> Mux/2
  cos(phi)/1 -> cos2(phi)/2
  Gain/1 -> Add2/2
  Constant2/1 -> Add4/2, Add2/1
  Add2/1 -> Product2/1
  Product2/1 -> Add3/4
  Gain1/1 -> Add4/1
  Add4/1 -> Product3/1
  Product3/1 -> Add3/3
  Product4/1 -> Gain2/1
  cos2(phi)/1 -> Product4/3
  Gain2/1 -> Add3/2
  Gain3/1 -> Divide1/1
  Divide1/1 -> Add3/1
  Add3/1 -> Divide2/1
  Divide2/1 -> g_z/2
  g_z/1 -> Mux/3
  g_x/1 -> Mux/1

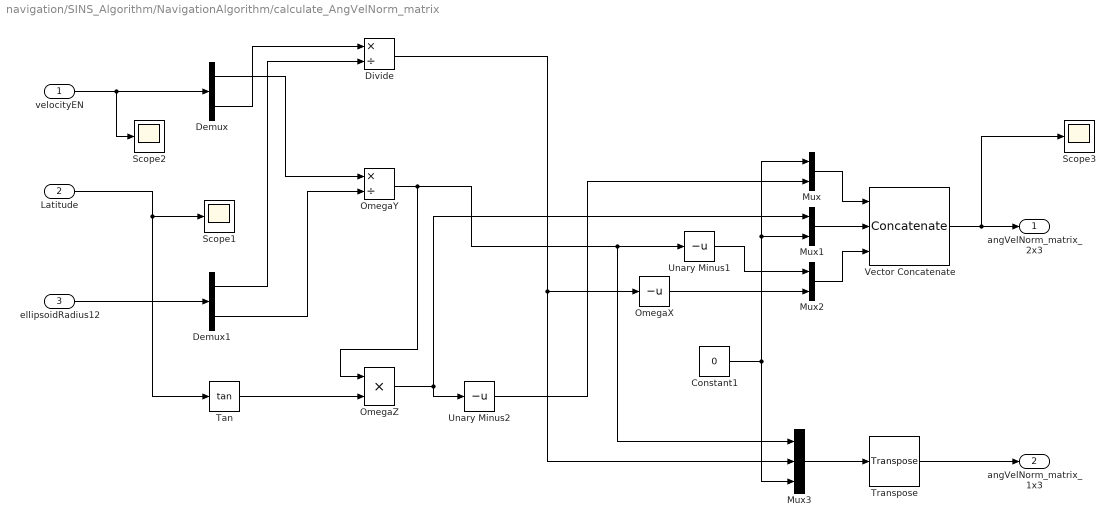
== system navigation/SINS_Algorithm/NavigationAlgorithm/calculate_AngVelNorm_matrix ==
  velocityEN : Inport
  Latitude : Inport  Port=2
  ellipsoidRadius12 : Inport  Port=3
  Constant1 : Constant  Value=0
  Demux : Demux  Outputs=2
  Demux1 : Demux  Outputs=2
  Divide : Product  Inputs=*/
  Mux : Mux  Inputs=2
  Mux1 : Mux  Inputs=2
  Mux2 : Mux  Inputs=2
  Mux3 : Mux  Inputs=3
  OmegaX : UnaryMinus
  OmegaY : Product  Inputs=*/
  OmegaZ : Product  Inputs=**
  Scope1 : Scope
  Scope2 : Scope
  Scope3 : Scope
  Tan : Trigonometry  Operator=tan
  Transpose : matrix_library/Transpose
      settings: SourceProductBaseCode=SL
  Unary Minus1 : UnaryMinus
  Unary Minus2 : UnaryMinus
  Vector Concatenate : Concatenate  NumInputs=3  Mode=Multidimensional array  ConcatenateDimension=2
  angVelNorm_matrix_2x3 : Outport
  angVelNorm_matrix_1x3 : Outport  Port=2
  wires:
  velocityEN/1 -> Scope2/1, Demux/1
  ellipsoidRadius12/1 -> Demux1/1
  Demux/2 -> Divide/1
  Demux1/1 -> Divide/2
  Divide/1 -> Mux3/2, OmegaX/1
  OmegaX/1 -> Mux2/2
  Demux/1 -> OmegaY/1
  Demux1/2 -> OmegaY/2
  OmegaY/1 -> OmegaZ/1, Mux3/1, Unary Minus1/1
  Unary Minus1/1 -> Mux2/1
  Tan/1 -> OmegaZ/2
  Latitude/1 -> Scope1/1, Tan/1
  OmegaZ/1 -> Unary Minus2/1, Mux1/1
  Unary Minus2/1 -> Mux/2
  Constant1/1 -> Mux3/3, Mux/1, Mux1/2
  Mux1/1 -> Vector Concatenate/2
  Mux/1 -> Vector Concatenate/1
  Mux2/1 -> Vector Concatenate/3
  Vector Concatenate/1 -> Scope3/1, angVelNorm_matrix_2x3/1
  Mux3/1 -> Transpose/1
  Transpose/1 -> angVelNorm_matrix_1x3/1

== system navigation/SINS_Algorithm/NavigationAlgorithm/calculate_AngVelNorm_matrix_3CH ==
  velocityENH : Inport
  Latitude : Inport  Port=2
  ellipsoidRadius12 : Inport  Port=3
  Constant : Constant  Value=0
  Create 3x3 Matrix : sharedutil/Create 3x3 Matrix  aMode=aMode
      settings: SourceProductBaseCode=AE,PW,DR,MT,UV,VE
  Demux : Demux  Outputs=3
  Demux1 : Demux  Outputs=2
  Divide : Product  Inputs=*/
  OmegaX : UnaryMinus
  OmegaY : Product  Inputs=*/
  OmegaZ : Product  Inputs=**/
  Tan : Trigonometry  Operator=tan
  Terminator : Terminator
  Unary Minus1 : UnaryMinus
  Unary Minus2 : UnaryMinus
  angVelNorm_matrix : Outport
  wires:
  velocityENH/1 -> Demux/1
  ellipsoidRadius12/1 -> Demux1/1
  Demux/2 -> Divide/1
  Demux1/1 -> Divide/2
  Divide/1 -> Create 3x3 Matrix/8, OmegaX/1
  OmegaX/1 -> Create 3x3 Matrix/6
  Demux/1 -> OmegaZ/1, OmegaY/1
  Demux1/2 -> OmegaZ/3, OmegaY/2
  OmegaY/1 -> Unary Minus1/1, Create 3x3 Matrix/7
  Unary Minus1/1 -> Create 3x3 Matrix/3
  Tan/1 -> OmegaZ/2
  Latitude/1 -> Tan/1
  OmegaZ/1 -> Unary Minus2/1, Create 3x3 Matrix/2
  Unary Minus2/1 -> Create 3x3 Matrix/4
  Constant/1 -> Create 3x3 Matrix/9, Create 3x3 Matrix/5, Create 3x3 Matrix/1
  Create 3x3 Matrix/1 -> angVelNorm_matrix/1
  Demux/3 -> Terminator/1

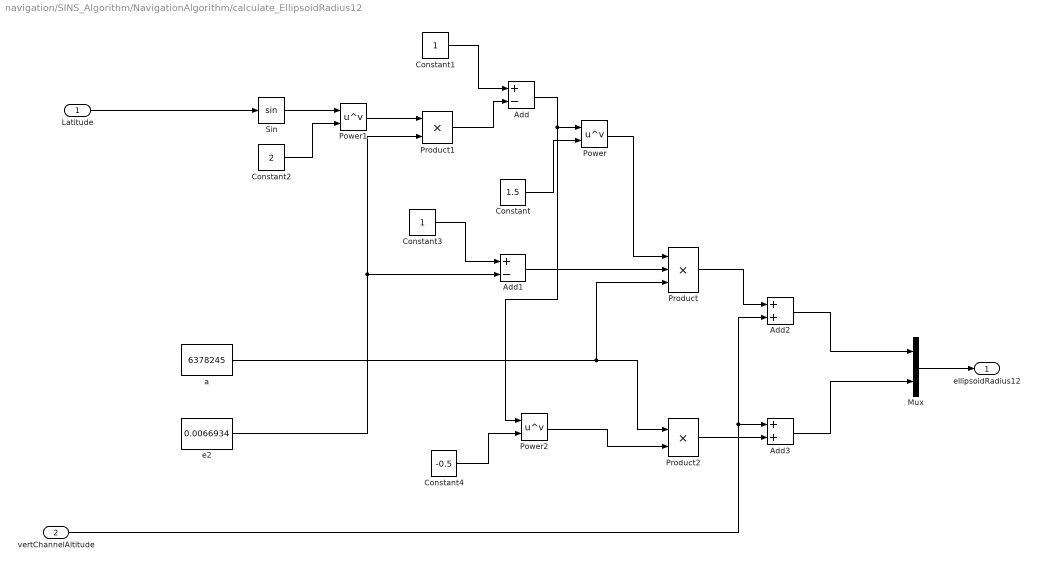
== system navigation/SINS_Algorithm/NavigationAlgorithm/calculate_EllipsoidRadius12 ==
  Latitude : Inport
  vertChannelAltitude : Inport  Port=2
  Add : Sum  Inputs=+-
  Add1 : Sum  Inputs=+-
  Add2 : Sum
  Add3 : Sum
  Constant : Constant  Value=1.5
  Constant1 : Constant
  Constant2 : Constant  Value=2
  Constant3 : Constant
  Constant4 : Constant  Value=-0.5
  Mux : Mux  Inputs=2
  Power : Math  Operator=pow  SaturateOnIntegerOverflow=on
  Power1 : Math  Operator=pow  SaturateOnIntegerOverflow=on
  Power2 : Math  Operator=pow  SaturateOnIntegerOverflow=on
  Product : Product  Inputs=3
  Product1 : Product
  Product2 : Product
  Sin : Trigonometry
  a : Constant  Value=6378245
  e2 : Constant  Value=0.0066934
  ellipsoidRadius12 : Outport
  wires:
  Mux/1 -> ellipsoidRadius12/1
  Constant1/1 -> Add/1
  Product1/1 -> Add/2
  Power1/1 -> Product1/1
  Sin/1 -> Power1/1
  Constant2/1 -> Power1/2
  Latitude/1 -> Sin/1
  e2/1 -> Add1/2, Product1/2
  Add/1 -> Power2/1, Power/1
  Constant/1 -> Power/2
  Power/1 -> Product/1
  Constant3/1 -> Add1/1
  Add1/1 -> Product/2
  a/1 -> Product2/1, Product/3
  Product/1 -> Add2/1
  vertChannelAltitude/1 -> Add2/2, Add3/1
  Add2/1 -> Mux/1
  Constant4/1 -> Power2/2
  Power2/1 -> Product2/2
  Product2/1 -> Add3/2
  Add3/1 -> Mux/2

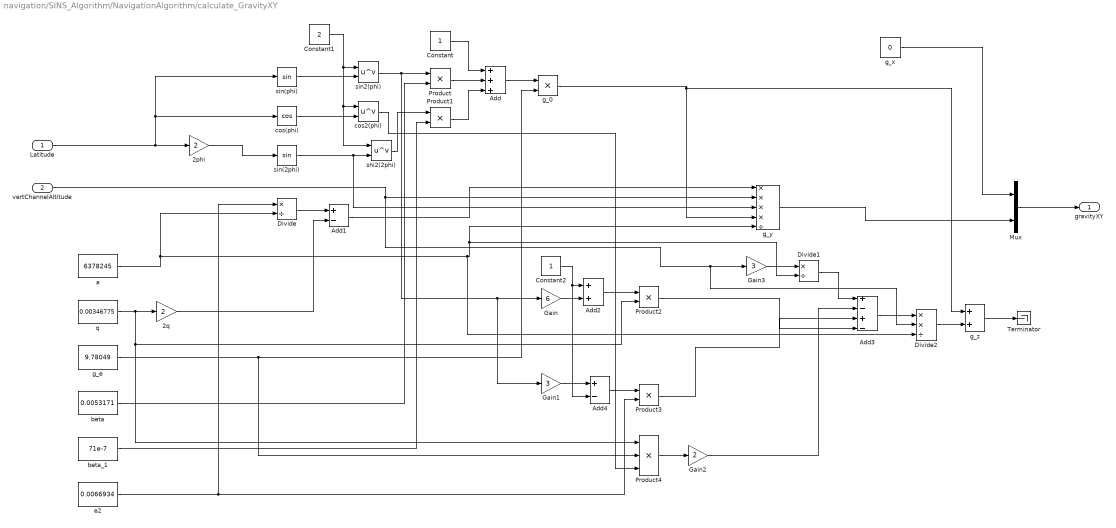
== system navigation/SINS_Algorithm/NavigationAlgorithm/calculate_GravityXY ==
  Latitude : Inport
  vertChannelAltitude : Inport  Port=2
  2phi : Gain  Gain=2
  2q : Gain  Gain=2
  Add : Sum  Inputs=+++
  Add1 : Sum  Inputs=+-
  Add2 : Sum
  Add3 : Sum  Inputs=+-+-
  Add4 : Sum  Inputs=+-
  Constant : Constant
  Constant1 : Constant  Value=2
  Constant2 : Constant
  Divide : Product  Inputs=*/
  Divide1 : Product  Inputs=*/
  Divide2 : Product  Inputs=**/
  Gain : Gain  Gain=6
  Gain1 : Gain  Gain=3
  Gain2 : Gain  Gain=2
  Gain3 : Gain  Gain=3
  Mux : Mux  Inputs=2
  Product{,1..3} (4 alike) : Product
  Product4 : Product  Inputs=3
  Terminator : Terminator
  a : Constant  Value=6378245
  beta : Constant  Value=0.0053171
  beta_1 : Constant  Value=71e-7
  cos(phi) : Trigonometry  Operator=cos
  cos2(phi) : Math  Operator=pow  SaturateOnIntegerOverflow=on
  e2 : Constant  Value=0.0066934
  g_0 : Product
  g_e : Constant  Value=9.78049
  g_x : Constant  Value=0
  g_y : Product  Inputs=****/
  g_z : Sum
  q : Constant  Value=0.00346775
  shi2(2phi) : Math  Operator=pow  SaturateOnIntegerOverflow=on
  sin(2phi) : Trigonometry
  sin(phi) : Trigonometry
  sin2(phi) : Math  Operator=pow  SaturateOnIntegerOverflow=on
  gravityXY : Outport
  wires:
  Mux/1 -> gravityXY/1
  Latitude/1 -> cos(phi)/1, sin(phi)/1, 2phi/1
  2phi/1 -> sin(2phi)/1
  sin(phi)/1 -> sin2(phi)/2
  Constant1/1 -> cos2(phi)/1, shi2(2phi)/1, sin2(phi)/1
  sin(2phi)/1 -> g_y/3, shi2(2phi)/2
  beta/1 -> Product/2
  sin2(phi)/1 -> Gain1/1, Gain/1, Product/1
  shi2(2phi)/1 -> Product1/1
  beta_1/1 -> Product1/2
  Product/1 -> Add/2
  Constant/1 -> Add/1
  Product1/1 -> Add/3
  Add/1 -> g_0/1
  g_e/1 -> Product4/2, g_0/2
  e2/1 -> Product3/2, Divide/1
  a/1 -> Divide2/3, Divide1/2, g_y/5, Divide/2
  Divide/1 -> Add1/1
  q/1 -> Product4/1, Product2/2, 2q/1
  2q/1 -> Add1/2
  Add1/1 -> g_y/1
  vertChannelAltitude/1 -> Divide2/2, Gain3/1, g_y/2
  g_0/1 -> g_z/1, g_y/4
  g_y/1 -> Mux/2
  cos(phi)/1 -> cos2(phi)/2
  Gain/1 -> Add2/2
  Constant2/1 -> Add4/2, Add2/1
  Add2/1 -> Product2/1
  Product2/1 -> Add3/4
  Gain1/1 -> Add4/1
  Add4/1 -> Product3/1
  Product3/1 -> Add3/3
  Product4/1 -> Gain2/1
  cos2(phi)/1 -> Product4/3
  Gain2/1 -> Add3/2
  Gain3/1 -> Divide1/1
  Divide1/1 -> Add3/1
  Add3/1 -> Divide2/1
  Divide2/1 -> g_z/2
  g_z/1 -> Terminator/1
  g_x/1 -> Mux/1

== system navigation/SINS_Algorithm/NavigationAlgorithm/calculate_U_matrix ==
  U_earth : Inport
  Latitude : Inport  Port=2
  Constant : Constant  Value=0
  Cos : Trigonometry  Operator=cos
  Mux : Mux  Inputs=2
  Mux1 : Mux  Inputs=2
  Mux2 : Mux  Inputs=2
  Mux3 : Mux  Inputs=3
  Product : Product
  Product1 : Product
  Sin : Trigonometry
  Transpose : matrix_library/Transpose
      settings: SourceProductBaseCode=SL
  Unary Minus : UnaryMinus
  Unary Minus1 : UnaryMinus
  Vector Concatenate : Concatenate  NumInputs=3  Mode=Multidimensional array  ConcatenateDimension=2
  U_matrix_2x3 : Outport
  U_matrix_1x3 : Outport  Port=2
  wires:
  Latitude/1 -> Sin/1, Cos/1
  U_earth/1 -> Product1/1, Product/1
  Cos/1 -> Product/2
  Product/1 -> Mux3/1, Unary Minus/1
  Unary Minus/1 -> Mux2/1
  Sin/1 -> Product1/2
  Product1/1 -> Mux1/1, Unary Minus1/1
  Unary Minus1/1 -> Mux/2
  Mux/1 -> Vector Concatenate/1
  Mux2/1 -> Vector Concatenate/3
  Mux1/1 -> Vector Concatenate/2
  Constant/1 -> Mux3/3, Mux3/2, Mux/1, Mux1/2, Mux2/2
  Vector Concatenate/1 -> U_matrix_2x3/1
  Mux3/1 -> Transpose/1
  Transpose/1 -> U_matrix_1x3/1

== system navigation/SINS_Algorithm/NavigationAlgorithm/calculate_U_matrix_3CH ==
  U_earth : Inport
  Latitude : Inport  Port=2
  Constant : Constant  Value=0
  Cos : Trigonometry  Operator=cos
  Create 3x3 Matrix : sharedutil/Create 3x3 Matrix  aMode=aMode
      settings: SourceProductBaseCode=AE,PW,DR,MT,UV,VE
  Product : Product
  Product1 : Product
  Sin : Trigonometry
  Unary Minus : UnaryMinus
  Unary Minus1 : UnaryMinus
  U_matrix : Outport
  wires:
  Latitude/1 -> Sin/1, Cos/1
  U_earth/1 -> Product1/1, Product/1
  Cos/1 -> Product/2
  Product/1 -> Unary Minus/1, Create 3x3 Matrix/7
  Unary Minus/1 -> Create 3x3 Matrix/3
  Sin/1 -> Product1/2
  Product1/1 -> Unary Minus1/1, Create 3x3 Matrix/2
  Unary Minus1/1 -> Create 3x3 Matrix/4
  Constant/1 -> Create 3x3 Matrix/9, Create 3x3 Matrix/8, Create 3x3 Matrix/6, Create 3x3 Matrix/5, Create 3x3 Matrix/1
  Create 3x3 Matrix/1 -> U_matrix/1

== system navigation/SINS_Algorithm/NavigationAlgorithm/eraseAccelZ ==
  accelerationXYZ : Inport
  Demux : Demux  Outputs=3
  Mux : Mux  Inputs=2
  Terminator : Terminator
  accelerationXY : Outport
  wires:
  accelerationXYZ/1 -> Demux/1
  Demux/1 -> Mux/1
  Demux/2 -> Mux/2
  Mux/1 -> accelerationXY/1
  Demux/3 -> Terminator/1
